simulink model "LKAS_AutoSave_DF_20220125_0841"  (R2018b)
settings: Solver=FixedStepDiscrete  StartTime=0.0  StopTime=10.0  FixedStep=0.01  RelTol=1e-3
InitFcn:
  | tmpVer = ver('MATLAB');
  | tmpVer = str2num(tmpVer.Version);
  | % -------------------------------------------------------------------
  | %  MATLAB file generated by Simulink.saveVars on 21-Nov-2019 10:06:14
  | %  MATLAB version: 7.13.0.564 (R2011b)
  | % -------------------------------------------------------------------
  | 
  | 
  | SInt16 = Simulink.AliasType;
  | SInt16.Description = 'Num';
  | if (tmpVer > 7.11)
  | 	SInt16.DataScope = 'Auto';
  | end
  | SInt16.HeaderFile = 'Rte_Type.h';
  | SInt16.BaseType = 'int16';
  | 
  | SInt32 = Simulink.AliasType;
  | SInt32.Description = 'Num';
  | if (tmpVer > 7.11)
  | 	SInt32.DataScope = 'Auto';
  | end
  | SInt32.HeaderFile = 'Rte_Type.h';
  | SInt32.BaseType = 'int32';
  | 
  | SInt8 = Simulink.AliasType;
  | SInt8.Description = 'Num';
  | if (tmpVer > 7.11)
  | 	SInt8.DataScope = 'Auto';
  | end
  | SInt8.HeaderFile = 'Rte_Type.h';
  | SInt8.BaseType = 'int8';
  | 
  | T_A_m2_1024_1_u32 = Simulink.NumericType;
  | T_A_m2_1024_1_u32.Description = 'm2 (square meters  (m2))';
  | if (tmpVer > 7.11)
  | 	T_A_m2_1024_1_u32.DataScope = 'Auto';
  | end
  | T_A_m2_1024_1_u32.HeaderFile = 'Rte_Type.h';
  | T_A_m2_1024_1_u32.DataTypeMode = 'Fixed-point: slope and bias scaling';
  | T_A_m2_1024_1_u32.SignednessBool = false;
  | T_A_m2_1024_1_u32.WordLength = 32;
  | T_A_m2_1024_1_u32.FixedExponent = -10;
  | T_A_m2_1024_1_u32.SlopeAdjustmentFactor = 1;
  | T_A_m2_1024_1_u32.Bias = 0;
  | T_A_m2_1024_1_u32.DataTypeOverride = 'Inherit';
  | T_A_m2_1024_1_u32.IsAlias = true;
  | 
  | T_A_m2_65536_1_u16 = Simulink.NumericType;
  | T_A_m2_65536_1_u16.Description = 'm2 (square meters  (m2))';
  | if (tmpVer > 7.11)
  | 	T_A_m2_65536_1_u16.DataScope = 'Auto';
  | end
  | T_A_m2_65536_1_u16.HeaderFile = 'Rte_Type.h';
  | T_A_m2_65536_1_u16.DataTypeMode = 'Fixed-point: slope and bias scaling';
  | T_A_m2_65536_1_u16.SignednessBool = false;
  | T_A_m2_65536_1_u16.WordLength = 16;
  | T_A_m2_65536_1_u16.FixedExponent = -16;
  | T_A_m2_65536_1_u16.SlopeAdjustmentFactor = 1;
  | T_A_m2_65536_1_u16.Bias = 0;
  | T_A_m2_65536_1_u16.DataTypeOverride = 'Inherit';
  | ... (+4647 lines)
StopFcn:
  | clear  T_A_m2_1024_1_u32 T_A_m2_65536_1_u16 T_A_m2_Float32 T_A_mm2_10_1_u16 T_A_mm2_4_1_s16 T_A_mm2_Float32 T_Cnt_Num_10_1_u32 T_Cnt_Num_1_1_s16 T_Cnt_Num_1_1_s32 T_Cnt_Num_1_1_s8 T_Cnt_Num_1_1_u16 T_Cnt_Num_1_1_u32 T_Cnt_Num_1_1_u8 T_E_J_1_1_s32 T_E_J_Float32 T_E_kJ_128_1_s32 T_E_kJ_Float32 T_E_kwh_10_1_u16 T_E_kwh_Float32 T_Epl_kwhpkm_100_1_u16 T_Epl_kwhpkm_Float32 T_F_N_1_1_s16 T_F_N_Float32 T_I_A_1000_1_u16 T_I_A_1048576_1_s32 T_I_A_2048_1_s16 T_I_A_32_1_s16 T_I_A_Float32 T_I_mA_1_1_s16 T_I_mA_32768_128_s16 T_I_mA_Float32 T_J_kgpm2_128_1_u16 T_J_kgpm2_Float32 T_K_NA_1000_1_s16 T_K_NA_100_1_s16 T_K_NA_100_1_u16 T_K_NA_1024_1_s16 T_K_NA_1024_1_u16 T_K_NA_128_1_s16 T_K_NA_128_1_u16 T_K_NA_128_1_u8 T_K_NA_16777216_1_u32 T_K_NA_16_1_s16 T_K_NA_16_1_u16 T_K_NA_16_1_u8 T_K_NA_1_16_u16 T_K_NA_1_1_s16 T_K_NA_1_1_u16 T_K_NA_1_1_u8 T_K_NA_32768_1_s16 T_K_NA_32768_1_u16 T_K_NA_32_1_s8 T_K_NA_4096_1_u16 T_K_NA_4194304_1_s32 T_K_NA_4194304_1_u16 T_K_NA_65536_1_s32 T_K_NA_65536_1_u16 T_K_NA_8192_1_s16 T_K_NA_8_1_s16 T_K_NA_Float32 T_M_Nm_16_1_s16 T_M_Nm_1_1_s16 T_M_Nm_32768_1_s16 T_M_Nm_32_1_s16 T_M_Nm_4_1_s16 T_M_Nm_512_1_s16 T_M_Nm_Float32 T_P_W_1_4_s16 T_P_W_1_8_s16 T_P_W_Float32 T_P_kW_128_1_s16 T_P_kW_1_8_s16 T_P_kW_8_1_s32 T_P_kW_Float32 T_Pct_pct_1024_1_s32 T_Pct_pct_1024_1_u32 T_Pct_pct_10_1_s16 T_Pct_pct_10_1_u32 T_Pct_pct_128_100_s8 T_Pct_pct_1_1_s16 T_Pct_pct_1_4_u8 T_Pct_pct_255_100_u16 T_Pct_pct_255_100_u8 T_Pct_pct_256_1_s16 T_Pct_pct_256_1_u16 T_Pct_pct_65535_100_u16 T_Pct_pct_Float32 T_R_ohm_1024_1_s16 T_R_ohm_32_1_s16 T_R_ohm_Float32 T_TK_K_16_1_s16 T_TK_K_Float32 T_T_degC_10_400_1_u16 T_T_degC_16_1_s16 T_T_degC_1_40_1_u8 T_T_degC_2_80_1_u8 T_T_degC_Float32 T_U_V_1000_1_u16 T_U_V_10_1_u8 T_U_V_200_1_u8 T_U_V_32_1_s16 T_U_V_4096_1_s16 T_U_V_512_1_s16 T_U_V_65535_8_u16 T_U_V_8192_1_u16 T_U_V_Float32 T_U_mV_1_1_s16 T_U_mV_256_20_u16 T_U_mV_Float32 T_V_l_256_1_s16 T_V_l_4096_1_s16 T_V_l_64_1_s16 T_V_l_65535_100_u16 T_V_l_Float32 T_V_ml_128_1_s16 T_V_ml_1_1_s16 T_V_ml_32768_1_s16 T_V_ml_Float32 T_V_ul_32_1_u16 T_V_ul_Float32 T_Vpl_clpkm_512_1_u16 T_Vpl_clpkm_Float32 T_a_kphps_16_1_s16 T_a_kphps_Float32 T_a_mps2_128_1_s16 T_a_mps2_Float32 T_c_MJpkg_256_1_s16 T_c_MJpkg_Float32 T_c_kJpgpK_1024_1_s16 T_c_kJpgpK_Float32 T_c_kJpkgpK_128_1_u16 T_c_kJpkgpK_Float32 T_chrg_Ah_1_1_s16 T_chrg_Ah_1_1_u16 T_chrg_Ah_1_1_u8 T_chrg_Ah_256_1_u16 T_chrg_Ah_4194304_1_s32 T_chrg_Ah_512_1_u16 T_chrg_Ah_8_1_u16 T_chrg_Ah_Float32 T_cmp_NA_100_1_s16 T_cmp_NA_128_1_s16 T_cmp_NA_16_1_s16 T_cmp_NA_32768_1_u16 T_cmp_NA_Float32 T_d2n_rpmps2_4_1_s16 T_d2n_rpmps2_Float32 T_dPct_pctps_16_1_s16 T_dPct_pctps_256_1_s16 T_dPct_pctps_Float32 T_dT_degCps_128_1_s16 T_dT_degCps_Float32 T_dV_lph_1_1_s16 T_dV_lph_Float32 T_dV_lpm_128_1_s16 T_dV_lpm_32_1_s16 T_dV_lpm_Float32 T_dV_lps_1024_1_u16 T_dV_lps_4_1_u16 T_dV_lps_Float32 T_dV_mlps_1024_1_s16 T_dV_mlps_Float32 T_d_BitField16 T_dm_gps_128_1_s16 T_dm_gps_128_1_u16 T_dm_gps_256_1_u16 T_dm_gps_Float32 T_dm_mgps_1_1_s16 T_dm_mgps_Float32 T_dn_rpmps_1_1_s16 T_dn_rpmps_2_1_s16 T_dn_rpmps_Float32 T_dp_Paps_1_1_s16 T_dp_Paps_Float32 T_dp_kPaps_1_1_s16 T_dp_kPaps_8_1_s16 T_dp_kPaps_Float32 T_dphi_degps_128_1_s16 T_dphi_degps_8_1_s16 T_dphi_degps_Float32 T_dr_ps_256_1_s16 T_dr_ps_Float32 T_drho_mgplps_1_2_s16 T_drho_mgplps_Float32 T_e_NA_1_1_u8 T_f_Hz_1_1_u16 T_f_Hz_1_1_u32 T_f_Hz_64_1_u16 T_f_Hz_8_1_s16 T_f_Hz_Float32 T_g_BitField32 T_l_km_16_1_s16 T_l_km_1_1_u16 T_l_km_1_1_u32 T_l_km_Float32 T_l_m_1024_1_s16 T_l_m_16_1_s16 T_l_m_1_1_u32 T_l_m_Float32 T_l_mm_16_1_s16 T_l_mm_1_1_u16 T_l_mm_4096_1_s16 T_l_mm_4_1_u8 T_l_mm_64_1_s16 T_l_mm_Float32 T_m_g_1_1_s16 T_m_g_2048_1_s16 T_m_g_32_1_u16 T_m_g_Float32 T_m_kg_1024_1_s16 T_m_kg_1_1_s16 T_m_kg_1_1_u32 T_m_kg_Float32 T_m_mg_128_1_s16 T_m_mg_32_1_s16 T_m_mg_Float32 T_n_rpm_1_1_s16 T_n_rpm_1_25_u8 T_n_rpm_256_50_u16 T_n_rpm_2_25_u8 T_n_rpm_4_1_u16 T_n_rpm_Float32 T_p_MPa_64_1_s16 T_p_MPa_Float32 T_p_Pa_1_1_s16 T_p_Pa_Float32 T_p_kPa_1_10_u16 T_p_kPa_1_1_s16 T_p_kPa_1_1_u8 T_p_kPa_256_1_u16 T_p_kPa_32_1_u16 T_p_kPa_64_1_s16 T_p_kPa_Float32 T_phi_deg_100_1_s16 T_phi_deg_1024_1_s16 T_phi_deg_128_1_s16 T_phi_deg_1_1_u8 T_phi_deg_256_1_s16 T_phi_deg_2_1_s8 T_phi_deg_32_1_s16 T_phi_deg_512_6_s32 T_phi_deg_Float32 T_phi_rad_2048_1_s16 T_phi_rad_Float32 T_r_NA_1024_1_s16 T_r_NA_1024_1_u16 T_r_NA_16384_1_s16 T_r_NA_16_1_s16 T_r_NA_256_1_s8 T_r_NA_256_1_u16 T_r_NA_32768_1_u16 T_r_NA_32_1_u16 T_r_NA_4096_1_s16 T_r_NA_65535_2_u16 T_r_NA_8192_1_u16 T_r_NA_Float32 T_rho_gpl_8192_1_s16 T_rho_gpl_Float32 T_rho_kgpm3_16_1_s16 T_rho_kgpm3_Float32 T_rho_mgpl_1_1_s16 T_rho_mgpl_64_1_s16 T_rho_mgpl_Float32 T_t_hour_1_1_s16 T_t_hour_Float32 T_t_m_1_1_u16 T_t_m_Float32 T_t_ms_1_1_s16 T_t_ms_1_1_u16 T_t_ms_1_1_u32 T_t_ms_4096_1_s16 T_t_ms_64_1_s16 T_t_ms_Float32 T_t_s_1000_1_s16 T_t_s_100_1_s16 T_t_s_10_1_s16 T_t_s_10_1_u16 T_t_s_1_1_s16 T_t_s_1_1_u16 T_t_s_1_1_u32 T_t_s_Float32 T_t_us_10_1_u32 T_t_us_1_1_s16 T_t_us_1_1_u32 T_t_us_1_4_u16 T_t_us_Float32 T_v_kph_1_1_u8 T_v_kph_64_1_s16 T_v_kph_64_1_u16 T_v_kph_Float32 T_v_mps_256_1_s16 T_v_mps_Float32 T_w_radps_32_1_s16 T_w_radps_Float32 T_y_BitField8 T_y_BitFieldDiagProgress T_y_BitFieldDiagStatus T_y_NA_1_1_u8 SInt16 SInt32 SInt8 T_BOOLEAN UInt16 UInt32 UInt8 s16 s32 s8 u16 u32 u8
model workspace (MAT data in the model file):
  MCOS : class17 (value not decoded)
  MCOS : class17 (value not decoded)
  MCOS : class17 (value not decoded)
  MCOS : class17 (value not decoded)
  MCOS : class17 (value not decoded)
  MCOS : class17 (value not decoded)
  MCOS : class17 (value not decoded)
  MCOS : class17 (value not decoded)
  MCOS : class17 (value not decoded)
  MCOS : class17 (value not decoded)
  MCOS : class17 (value not decoded)
  MCOS : class17 (value not decoded)
  MCOS : class17 (value not decoded)
  MCOS : class17 (value not decoded)
  MCOS : class17 (value not decoded)
  MCOS : class17 (value not decoded)
  MCOS : class17 (value not decoded)
  MCOS : class17 (value not decoded)
  MCOS : class17 (value not decoded)
  MCOS : class17 (value not decoded)
  MCOS : class17 (value not decoded)
  MCOS : class17 (value not decoded)
  MCOS : class17 (value not decoded)
  MCOS : class17 (value not decoded)
  MCOS : class17 (value not decoded)
  MCOS : class17 (value not decoded)
  MCOS : class17 (value not decoded)
  MCOS : class17 (value not decoded)
  MCOS : class17 (value not decoded)
  MCOS : class17 (value not decoded)
  MCOS : class17 (value not decoded)
  MCOS : class17 (value not decoded)
  MCOS : class17 (value not decoded)
  MCOS : class17 (value not decoded)
  MCOS : class17 (value not decoded)
  MCOS : class17 (value not decoded)
  MCOS : class17 (value not decoded)
  MCOS : class17 (value not decoded)
  MCOS : class17 (value not decoded)
  MCOS : class17 (value not decoded)
  MCOS : class17 (value not decoded)
  MCOS : class17 (value not decoded)
  MCOS : class17 (value not decoded)
  MCOS : class17 (value not decoded)
  MCOS : class17 (value not decoded)
  MCOS : class17 (value not decoded)
  MCOS : class17 (value not decoded)
  MCOS : class17 (value not decoded)
  MCOS : class17 (value not decoded)
  MCOS : class17 (value not decoded)
  MCOS : class17 (value not decoded)
  MCOS : class17 (value not decoded)
  MCOS : class17 (value not decoded)
  MCOS : class17 (value not decoded)
  MCOS : class17 (value not decoded)
  MCOS : class17 (value not decoded)
  MCOS : class17 (value not decoded)
  MCOS : class17 (value not decoded)
  MCOS : class17 (value not decoded)
  MCOS : class17 (value not decoded)
  MCOS : class17 (value not decoded)
  MCOS : class17 (value not decoded)
  MCOS : class17 (value not decoded)
  MCOS : class17 (value not decoded)
  MCOS : class17 (value not decoded)
  MCOS : class17 (value not decoded)
  MCOS : class17 (value not decoded)
  MCOS : class17 (value not decoded)
  MCOS : class17 (value not decoded)
  MCOS : class17 (value not decoded)
  MCOS : class17 (value not decoded)
  MCOS : class17 (value not decoded)
  MCOS : class17 (value not decoded)
  MCOS : class17 (value not decoded)
  MCOS : class17 (value not decoded)
  MCOS : class17 (value not decoded)
  MCOS : class17 (value not decoded)
  MCOS : class17 (value not decoded)
  MCOS : class17 (value not decoded)
  MCOS : class17 (value not decoded)
  MCOS : class17 (value not decoded)
  MCOS : class17 (value not decoded)
  MCOS : class17 (value not decoded)
  MCOS : class17 (value not decoded)
  MCOS : class17 (value not decoded)
  MCOS : class17 (value not decoded)
  MCOS : class17 (value not decoded)
  MCOS : class17 (value not decoded)
  MCOS : class17 (value not decoded)
  MCOS : class17 (value not decoded)
  MCOS : class17 (value not decoded)
  MCOS : class17 (value not decoded)
  MCOS : class17 (value not decoded)
  MCOS : class17 (value not decoded)
  MCOS : class17 (value not decoded)
  MCOS : class17 (value not decoded)
  MCOS : class17 (value not decoded)
  MCOS : class17 (value not decoded)
  MCOS : class17 (value not decoded)
  MCOS : class17 (value not decoded)
  MCOS : class17 (value not decoded)
  MCOS : class17 (value not decoded)
undefined symbols (not defined in the file): LKA_CarWidth, LKA_SampleTime, LKA_StrRatio_C, LKA_Veh2CamL_C, LKA_Veh2CamW_C, LKA_WhlBaseL_C, LL_CompHdAg_C, LL_CompSWA_C, LL_CrvtPrvwT_C, LL_DesDvt_C, LL_DvtComp_C, LL_DvtPrvwT_C, LL_DvtSpdDet_vDvtSpdMin_C, LL_HandsOff_ExitTime, LL_HandsOff_TextTime, LL_HandsOff_WarnTime, LL_HdAgExT_C, LL_HdAgPrvwT_C, LL_LAccMax_C, LL_LAccRMax_C, LL_LDW_EarliestWarnLine_C, LL_LDW_LatestWarnLine_C, LL_LDWS_SUPPRESS_HEADING, LL_LFClb_TFC_FfCtlRatio_C, LL_LFClb_TFC_KdBalance_C, LL_LFClb_TFC_KdMaxSWA_C, LL_LFClb_TFC_KdV1_C, LL_LFClb_TFC_KdV2_C, LL_LFClb_TFC_KdVehSpdLwr_C, LL_LFClb_TFC_KdVehSpdUpr_C, LL_LFClb_TFC_Ki_C, LL_LFClb_TFC_KiMaxSWA_C, LL_LFClb_TFC_Kp_C, LL_LFClb_TFC_KpKlat_C, LL_LFClb_TFC_KpV1_C, LL_LFClb_TFC_KpV2_C, LL_LFClb_TFC_KpVehSpdLwr_C, LL_LFClb_TFC_KpVehSpdUpr_C, LL_LFClb_TFC_PrvwT_C, LL_LKA_EarliestWarnLine_C, LL_LKA_LatestWarnLine_C, LL_LKAExPrcs_ExitC0Dvt, LL_LKAExPrcs_ExitC0Swt, LL_LKAExPrcs_tiExitTime1, LL_LKAExPrcs_tiExitTime2, LL_LKAExPrcs_tiExitTime3, LL_LKAS_OUT_OF_CONTROL_LAT_VEL, LL_LKAS_OUT_OF_CONTROL_TTLC, LL_LKASWASyn_M0, LL_LKASWASyn_M1, LL_LKASWASyn_M2, LL_LKASWASyn_M3K, LL_LKASWASyn_SWAaddMax, LL_LKASWASyn_T2, LL_LKASWASyn_tiTrqSwaRtTime, LL_LKASWASyn_tiTrqSwaTime, LL_LKASWASyn_TrqMax, LL_LKASWASyn_TrqSwaAddSwt, LL_LKASWASyn_TrqSwaRateDiff, LL_LSpdCompT_C ... (+43)
libraries: simulink x136, canmsglib x8, dspstat3 x3, simulink_extras x1
(part 5 of 20)

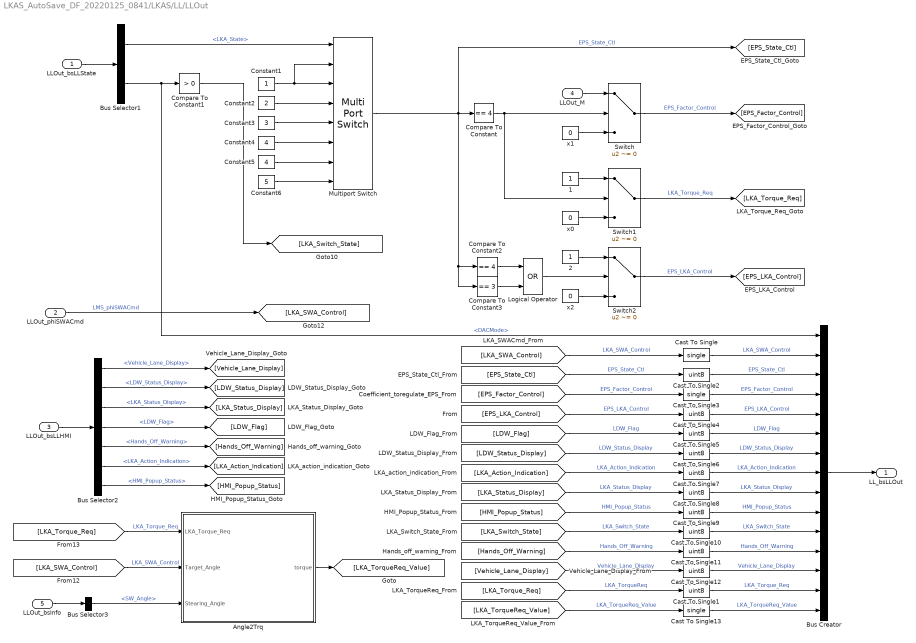
== system LKAS_AutoSave_DF_20220125_0841/LKAS/LL/LLOut ==
  LLOut_bsLLState : Inport
  LLOut_phiSWACmd : Inport  Port=2
  LLOut_bsLLHMI : Inport  Port=3
  LLOut_M : Inport  Port=4
  LLOut_bsInfo : Inport  Port=5
  1 : Constant  OutDataTypeStr=uint8
      settings: AttributesFormatString=DT: %<OutDataTypeStr>
  2 : Constant  OutDataTypeStr=uint8
      settings: AttributesFormatString=DT: %<OutDataTypeStr>
  Angle2Trq : Subsystem
  Bus Creator : BusCreator  Inputs=15
  Bus Selector1 : BusSelector  OutputSignals=LKA_State,DACMode
  Bus Selector2 : BusSelector  OutputSignals=Vehicle_Lane_Display,LDW_Status_Display,LKA_Status_Display,LDW_Flag,Hands_Off_Warning,LKA_Action_Indication,HMI_Popup_Status
  Bus Selector3 : BusSelector  OutputSignals=bsSWAInfo.SW_Angle
  Cast To Single : DataTypeConversion  OutDataTypeStr=single
  Cast To Single{1..2,4..12} (11 alike) : DataTypeConversion  OutDataTypeStr=uint8
  Cast To Single13 : DataTypeConversion  OutDataTypeStr=single
  Cast To Single3 : DataTypeConversion  OutDataTypeStr=single
  Compare To Constant : simulink/Logic and Bit Operations/Compare To Constant  relop===  const=4  OutDataTypeStr=boolean
  Compare To Constant1 : simulink/Logic and Bit Operations/Compare To Constant  relop=>  const=0  OutDataTypeStr=boolean
  Compare To Constant2 : simulink/Logic and Bit Operations/Compare To Constant  relop===  const=4  OutDataTypeStr=boolean
  Compare To Constant3 : simulink/Logic and Bit Operations/Compare To Constant  relop===  const=3  OutDataTypeStr=boolean
  Constant1 : Constant  OutDataTypeStr=uint8
  Constant2 : Constant  Value=2  OutDataTypeStr=uint8
  Constant3 : Constant  Value=3  OutDataTypeStr=uint8
  Constant4 : Constant  Value=4  OutDataTypeStr=uint8
  Constant5 : Constant  Value=4  OutDataTypeStr=uint8
  Constant6 : Constant  Value=5  OutDataTypeStr=uint8
  Logical Operator : Logic  Operator=OR  AllPortsSameDT=off  OutDataTypeStr=boolean
  Multiport Switch : MultiPortSwitch  DataPortOrder=Zero-based contiguous  Inputs=7  zeroidx=on
  Switch : Switch  Criteria=u2 ~= 0
      settings: AttributesFormatString=%<Criteria>
  Switch1 : Switch  Criteria=u2 ~= 0
      settings: AttributesFormatString=%<Criteria>
  Switch2 : Switch  Criteria=u2 ~= 0
      settings: AttributesFormatString=%<Criteria>
  x0 : Constant  Value=0  OutDataTypeStr=uint8
      settings: AttributesFormatString=DT: %<OutDataTypeStr>
  x1 : Constant  Value=0  OutDataTypeStr=uint8
      settings: AttributesFormatString=DT: %<OutDataTypeStr>
  x2 : Constant  Value=0  OutDataTypeStr=uint8
      settings: AttributesFormatString=DT: %<OutDataTypeStr>
  LL_bsLLOut : Outport
      settings: AttributesFormatString=Disable Action: %<OutputWhenDisabled>
  wires:
  Cast To Single13/1 -> Bus Creator/15  "LKA_TorqueReq_Value"
  [LKA_TorqueReq_Value] -> Cast To Single13/1  "LKA_TorqueReq_Value"
  Cast To Single1/1 -> Bus Creator/14  "LKA_Torque_Req"
  [LKA_Torque_Req] -> Cast To Single1/1  "LKA_TorqueReq"
  Cast To Single7/1 -> Bus Creator/8  "LKA_Action_Indication"
  Compare To Constant/1 -> Switch/2, Switch1/2
  [Vehicle_Lane_Display] -> Cast To Single12/1  "Vehicle_Lane_Display"
  [EPS_LKA_Control] -> Cast To Single4/1  "EPS_LKA_Control"
  [LDW_Flag] -> Cast To Single5/1  "LDW_Flag"
  [EPS_Factor_Control] -> Cast To Single3/1  "EPS_Factor_Control"
  [LKA_Action_Indication] -> Cast To Single7/1  "LKA_Action_Indication"
  Constant6/1 -> Multiport Switch/8
  Cast To Single5/1 -> Bus Creator/6  "LDW_Flag"
  [HMI_Popup_Status] -> Cast To Single9/1  "HMI_Popup_Status"
  Bus Selector1/1 -> Multiport Switch/1  "<LKA_State>"
  [LKA_Status_Display] -> Cast To Single8/1  "LKA_Status_Display"
  [LKA_SWA_Control] -> Cast To Single/1  "LKA_SWA_Control"
  Cast To Single/1 -> Bus Creator/2  "LKA_SWA_Control"
  [LDW_Status_Display] -> Cast To Single6/1  "LDW_Status_Display"
  [LKA_Switch_State] -> Cast To Single10/1  "LKA_Switch_State"
  [Hands_Off_Warning] -> Cast To Single11/1  "Hands_Off_Warning"
  Cast To Single8/1 -> Bus Creator/9  "LKA_Status_Display"
  Cast To Single4/1 -> Bus Creator/5  "EPS_LKA_Control"
  Cast To Single10/1 -> Bus Creator/11  "LKA_Switch_State"
  Bus Selector1/2 -> Bus Creator/1, Compare To Constant1/1  "<DACMode>"
  Constant2/1 -> Multiport Switch/4
  Cast To Single2/1 -> Bus Creator/3  "EPS_State_Ctl"
  Bus Creator/1 -> LL_bsLLOut/1
  Cast To Single3/1 -> Bus Creator/4  "EPS_Factor_Control"
  Constant3/1 -> Multiport Switch/5
  Multiport Switch/1 -> Compare To Constant2/1, Compare To Constant3/1, [EPS_State_Ctl], Compare To Constant/1  "EPS_State_Ctl"
  Switch/1 -> [EPS_Factor_Control]  "EPS_Factor_Control"
  Cast To Single6/1 -> Bus Creator/7  "LDW_Status_Display"
  Cast To Single12/1 -> Bus Creator/13  "Vehicle_Lane_Display"
  [EPS_State_Ctl] -> Cast To Single2/1  "EPS_State_Ctl"
  LLOut_bsLLState/1 -> Bus Selector1/1
  Compare To Constant1/1 -> [LKA_Switch_State]
  Constant4/1 -> Multiport Switch/6
  Cast To Single9/1 -> Bus Creator/10  "HMI_Popup_Status"
  LLOut_M/1 -> Switch/1
  Cast To Single11/1 -> Bus Creator/12  "Hands_Off_Warning"
  Constant5/1 -> Multiport Switch/7
  Constant1/1 -> Multiport Switch/2, Multiport Switch/3
  Bus Selector2/5 -> [Hands_Off_Warning]  "<Hands_Off_Warning>"
  Bus Selector2/6 -> [LKA_Action_Indication]  "<LKA_Action_Indication>"
  Bus Selector2/2 -> [LDW_Status_Display]  "<LDW_Status_Display>"
  LLOut_bsLLHMI/1 -> Bus Selector2/1
  Bus Selector2/4 -> [LDW_Flag]  "<LDW_Flag>"
  Bus Selector2/3 -> [LKA_Status_Display]  "<LKA_Status_Display>"
  Bus Selector2/7 -> [HMI_Popup_Status]  "<HMI_Popup_Status>"
  Bus Selector2/1 -> [Vehicle_Lane_Display]  "<Vehicle_Lane_Display>"
  Switch1/1 -> [LKA_Torque_Req]  "LKA_Torque_Req"
  1/1 -> Switch1/1
  x0/1 -> Switch1/3
  LLOut_phiSWACmd/1 -> [LKA_SWA_Control]  "LMS_phiSWACmd"
  [LKA_Torque_Req] -> Angle2Trq/1(LKA_Torque_Req)  "LKA_Torque_Req"
  [LKA_SWA_Control] -> Angle2Trq/2(Target_Angle)  "LKA_SWA_Control"
  Angle2Trq/1(torque) -> [LKA_TorqueReq_Value]
  LLOut_bsInfo/1 -> Bus Selector3/1
  Bus Selector3/1 -> Angle2Trq/3(Stearing_Angle)  "<SW_Angle>"
  x1/1 -> Switch/3
  Compare To Constant2/1 -> Logical Operator/1
  Compare To Constant3/1 -> Logical Operator/2
  Logical Operator/1 -> Switch2/2
  Switch2/1 -> [EPS_LKA_Control]  "EPS_LKA_Control"
  2/1 -> Switch2/1
  x2/1 -> Switch2/3

== system LKAS_AutoSave_DF_20220125_0841/LKAS/LLClb/ConstantClb ==
  Bus Creator : BusCreator  Inputs=6
  Data Type Conversion{2..4,6,13,22} (6 alike) : DataTypeConversion  OutDataTypeStr=single
  LKA_CarWidth=1.8 : Constant  Value=LKA_CarWidth
  LKA_SampleTime=0.01 : Constant  Value=LKA_SampleTime  OutDataTypeStr=single
  LKA_StrRatio_C=15.3 : Constant  Value=LKA_StrRatio_C
  LKA_Veh2CamL_C=1.56 : Constant  Value=LKA_Veh2CamL_C
  LKA_Veh2CamW_C=0.9 : Constant  Value=LKA_Veh2CamW_C  OutDataTypeStr=single
  LKA_WhlBaseL_C=2.65 : Constant  Value=LKA_WhlBaseL_C
  Switch{,1..3,11,19} (6 alike) : Switch  Criteria=u2 ~= 0  OutDataTypeStr=single
  ConstantClb : Outport
  wires:
  LKA_SampleTime=0.01/1 -> Switch19/3  "LKA_SampleTime"
  Data Type Conversion3/1 -> Switch19/1, Switch19/2
  Switch19/1 -> Bus Creator/1  "LKA_SampleTime"
  Switch2/1 -> Bus Creator/4  "LKA_WhlBaseL_C"
  Switch/1 -> Bus Creator/2  "LKA_Veh2CamW_C"
  Switch1/1 -> Bus Creator/3  "LKA_Veh2CamL_C"
  Switch11/1 -> Bus Creator/6  "LKA_CarWidth"
  Switch3/1 -> Bus Creator/5  "LKA_StrRatio_C"
  Bus Creator/1 -> ConstantClb/1
  LKA_CarWidth=1.8/1 -> Switch11/3  "LKA_CarWidth"
  Data Type Conversion22/1 -> Switch11/2, Switch11/1
  LKA_StrRatio_C=15.3/1 -> Switch3/3  "LKA_StrRatio_C"
  Data Type Conversion6/1 -> Switch3/2, Switch3/1
  Data Type Conversion4/1 -> Switch2/2, Switch2/1
  LKA_WhlBaseL_C=2.65/1 -> Switch2/3  "LKA_WhlBaseL_C"
  LKA_Veh2CamL_C=1.56/1 -> Switch1/3  "LKA_Veh2CamL_C"
  Data Type Conversion2/1 -> Switch1/2, Switch1/1
  Data Type Conversion13/1 -> Switch/2, Switch/1
  LKA_Veh2CamW_C=0.9/1 -> Switch/3  "LKA_Veh2CamW_C"

== system LKAS_AutoSave_DF_20220125_0841/LKAS/LLClb/LDWClb ==
  Bus Creator : BusCreator  Inputs=1
  Data Type Conversion6 : DataTypeConversion  OutDataTypeStr=single
  LL_LDWS_SUPPRESS_HEADING=2 : Constant  Value=LL_LDWS_SUPPRESS_HEADING  OutDataTypeStr=single
  Switch2 : Switch  Criteria=u2 ~= 0  OutDataTypeStr=single
  LDWClb : Outport
  wires:
  Data Type Conversion6/1 -> Switch2/2, Switch2/1
  LL_LDWS_SUPPRESS_HEADING=2/1 -> Switch2/3
  Switch2/1 -> Bus Creator/1  "LL_LDWS_SUPPRESS_HEADING"
  Bus Creator/1 -> LDWClb/1

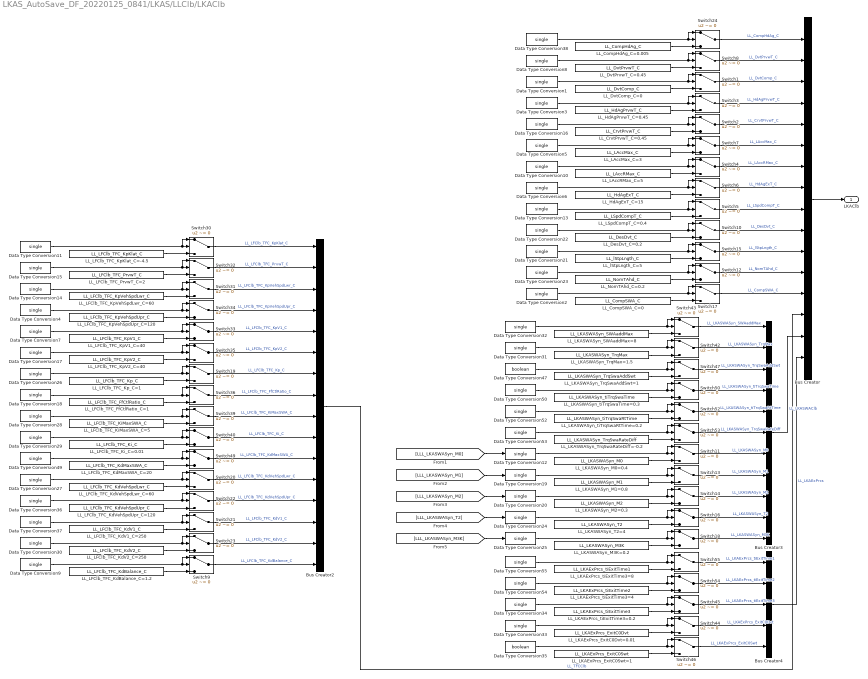
== system LKAS_AutoSave_DF_20220125_0841/LKAS/LLClb/LKAClb ==
  Bus Creator : BusCreator  Inputs=16
  Bus Creator2 : BusCreator  Inputs=16
  Bus Creator3 : BusCreator  Inputs=11
  Bus Creator4 : BusCreator  Inputs=5
  Data Type Conversion{1..34,36..38,49..50,52..55} (43 alike) : DataTypeConversion  OutDataTypeStr=single
  Data Type Conversion35 : DataTypeConversion  OutDataTypeStr=boolean
  Data Type Conversion47 : DataTypeConversion  OutDataTypeStr=boolean
  LL_CompHdAg_C=0.005 : Constant  Value=LL_CompHdAg_C  OutDataTypeStr=single
  LL_CompSWA_C=0 : Constant  Value=LL_CompSWA_C  OutDataTypeStr=single
  LL_CrvtPrvwT_C=0.45 : Constant  Value=LL_CrvtPrvwT_C  OutDataTypeStr=single
  LL_DesDvt_C=0.2 : Constant  Value=LL_DesDvt_C  OutDataTypeStr=single
  LL_DvtComp_C=0 : Constant  Value=LL_DvtComp_C  OutDataTypeStr=single
  LL_DvtPrvwT_C=0.45 : Constant  Value=LL_DvtPrvwT_C  OutDataTypeStr=single
  LL_HdAgExT_C=15 : Constant  Value=LL_HdAgExT_C  OutDataTypeStr=single
  LL_HdAgPrvwT_C=0.45 : Constant  Value=LL_HdAgPrvwT_C  OutDataTypeStr=single
  LL_LAccMax_C=3 : Constant  Value=LL_LAccMax_C  OutDataTypeStr=single
  LL_LAccRMax_C=5 : Constant  Value=LL_LAccRMax_C  OutDataTypeStr=single
  LL_LFClb_TFC_FfCtlRatio_C=1 : Constant  Value=LL_LFClb_TFC_FfCtlRatio_C  OutDataTypeStr=single
  LL_LFClb_TFC_KdBalance_C=1.2 : Constant  Value=LL_LFClb_TFC_KdBalance_C  OutDataTypeStr=single
  LL_LFClb_TFC_KdMaxSWA_C=20 : Constant  Value=LL_LFClb_TFC_KdMaxSWA_C  OutDataTypeStr=single
  LL_LFClb_TFC_KdV1_C=250 : Constant  Value=LL_LFClb_TFC_KdV1_C  OutDataTypeStr=single
  LL_LFClb_TFC_KdV2_C=250 : Constant  Value=LL_LFClb_TFC_KdV2_C  OutDataTypeStr=single
  LL_LFClb_TFC_KdVehSpdLwr_C=60 : Constant  Value=LL_LFClb_TFC_KdVehSpdLwr_C  OutDataTypeStr=single
  LL_LFClb_TFC_KdVehSpdUpr_C=120 : Constant  Value=LL_LFClb_TFC_KdVehSpdUpr_C  OutDataTypeStr=single
  LL_LFClb_TFC_KiMaxSWA_C=5 : Constant  Value=LL_LFClb_TFC_KiMaxSWA_C  OutDataTypeStr=single
  LL_LFClb_TFC_Ki_C=0.01 : Constant  Value=LL_LFClb_TFC_Ki_C  OutDataTypeStr=single
  LL_LFClb_TFC_KpKlat_C=-4.5 : Constant  Value=LL_LFClb_TFC_KpKlat_C  OutDataTypeStr=single
  LL_LFClb_TFC_KpV1_C=40 : Constant  Value=LL_LFClb_TFC_KpV1_C  OutDataTypeStr=single
  LL_LFClb_TFC_KpV2_C=40 : Constant  Value=LL_LFClb_TFC_KpV2_C  OutDataTypeStr=single
  LL_LFClb_TFC_KpVehSpdLwr_C=60 : Constant  Value=LL_LFClb_TFC_KpVehSpdLwr_C  OutDataTypeStr=single
  LL_LFClb_TFC_KpVehSpdUpr_C=120 : Constant  Value=LL_LFClb_TFC_KpVehSpdUpr_C  OutDataTypeStr=single
  LL_LFClb_TFC_Kp_C=1 : Constant  Value=LL_LFClb_TFC_Kp_C  OutDataTypeStr=single
  LL_LFClb_TFC_PrvwT_C=2 : Constant  Value=LL_LFClb_TFC_PrvwT_C  OutDataTypeStr=single
  LL_LKAExPrcs_ExitC0Dvt=0.01 : Constant  Value=LL_LKAExPrcs_ExitC0Dvt  OutDataTypeStr=single
  LL_LKAExPrcs_ExitC0Swt=1 : Constant  Value=LL_LKAExPrcs_ExitC0Swt  OutDataTypeStr=boolean
  LL_LKAExPrcs_tiExitTime3=0.2 : Constant  Value=LL_LKAExPrcs_tiExitTime3  OutDataTypeStr=single
  LL_LKAExPrcs_tiExitTime3=4 : Constant  Value=LL_LKAExPrcs_tiExitTime2  OutDataTypeStr=single
  LL_LKAExPrcs_tiExitTime3=8 : Constant  Value=LL_LKAExPrcs_tiExitTime1  OutDataTypeStr=single
  LL_LKASWASyn_M0=0.4 : Constant  Value=LL_LKASWASyn_M0  OutDataTypeStr=single
  LL_LKASWASyn_M1=0.8 : Constant  Value=LL_LKASWASyn_M1  OutDataTypeStr=single
  LL_LKASWASyn_M2=0.3 : Constant  Value=LL_LKASWASyn_M2  OutDataTypeStr=single
  LL_LKASWASyn_M3K=0.2 : Constant  Value=LL_LKASWASyn_M3K  OutDataTypeStr=single
  LL_LKASWASyn_SWAaddMax=8 : Constant  Value=LL_LKASWASyn_SWAaddMax  OutDataTypeStr=single
  LL_LKASWASyn_T2=4 : Constant  Value=LL_LKASWASyn_T2  OutDataTypeStr=single
  LL_LKASWASyn_TrqMax=1.5 : Constant  Value=LL_LKASWASyn_TrqMax  OutDataTypeStr=single
  LL_LKASWASyn_TrqSwaAddSwt=1 : Constant  Value=LL_LKASWASyn_TrqSwaAddSwt  OutDataTypeStr=boolean
  LL_LKASWASyn_TrqSwaRateDiff=-0.2 : Constant  Value=LL_LKASWASyn_TrqSwaRateDiff  OutDataTypeStr=single
  LL_LKASWASyn_tiTrqSwaRtTime=0.2 : Constant  Value=LL_LKASWASyn_tiTrqSwaRtTime  OutDataTypeStr=single
  LL_LKASWASyn_tiTrqSwaTime=0.3 : Constant  Value=LL_LKASWASyn_tiTrqSwaTime  OutDataTypeStr=single
  LL_LSpdCompT_C=0.4 : Constant  Value=LL_LSpdCompT_C  OutDataTypeStr=single
  LL_NomTAhd_C=0.2 : Constant  Value=LL_NomTAhd_C  OutDataTypeStr=single
  LL_lStpLngth_C=5 : Constant  Value=LL_lStpLngth_C  OutDataTypeStr=single
  Switch{1..24,30..36,39..40,42..45,49..50,52..55} (43 alike) : Switch  Criteria=u2 ~= 0  OutDataTypeStr=single
  Switch46 : Switch  Criteria=u2 ~= 0  OutDataTypeStr=boolean
  Switch47 : Switch  Criteria=u2 ~= 0  OutDataTypeStr=boolean
  LKAClb : Outport
  wires:
  [LLL_LKASWASyn_M3K] -> Data Type Conversion25/1
  Switch18/1 -> Bus Creator3/11  "LL_LKASWASyn_M3K"
  LL_LKASWASyn_M3K=0.2/1 -> Switch18/3
  Data Type Conversion25/1 -> Switch18/1, Switch18/2
  [LLL_LKASWASyn_M0] -> Data Type Conversion12/1
  Switch11/1 -> Bus Creator3/7  "LL_LKASWASyn_M0"
  LL_LKASWASyn_M0=0.4/1 -> Switch11/3
  Data Type Conversion12/1 -> Switch11/1, Switch11/2
  Data Type Conversion19/1 -> Switch13/2, Switch13/1
  LL_LKASWASyn_M1=0.8/1 -> Switch13/3
  Switch13/1 -> Bus Creator3/8  "LL_LKASWASyn_M1"
  [LLL_LKASWASyn_M1] -> Data Type Conversion19/1
  [LLL_LKASWASyn_M2] -> Data Type Conversion20/1
  Switch14/1 -> Bus Creator3/9  "LL_LKASWASyn_M2"
  LL_LKASWASyn_M2=0.3/1 -> Switch14/3
  Data Type Conversion20/1 -> Switch14/1, Switch14/2
  Data Type Conversion24/1 -> Switch16/2, Switch16/1
  LL_LKASWASyn_T2=4/1 -> Switch16/3
  Switch16/1 -> Bus Creator3/10  "LL_LKASWASyn_T2"
  [LLL_LKASWASyn_T2] -> Data Type Conversion24/1
  Data Type Conversion9/1 -> Switch9/2, Switch9/1
  LL_LFClb_TFC_KdBalance_C=1.2/1 -> Switch9/3
  Switch9/1 -> Bus Creator2/16  "LL_LFClb_TFC_KdBalance_C"
  LL_LKAExPrcs_tiExitTime3=8/1 -> Switch55/3
  Data Type Conversion55/1 -> Switch55/1, Switch55/2
  Switch55/1 -> Bus Creator4/1  "LL_LKAExPrcs_tiExitTime1"
  Switch54/1 -> Bus Creator4/2  "LL_LKAExPrcs_tiExitTime2"
  Data Type Conversion54/1 -> Switch54/2, Switch54/1
  LL_LKAExPrcs_tiExitTime3=4/1 -> Switch54/3
  Switch53/1 -> Bus Creator3/6  "LL_LKASWASyn_TrqSwaRateDiff"
  LL_LKASWASyn_TrqSwaRateDiff=-0.2/1 -> Switch53/3
  Data Type Conversion53/1 -> Switch53/1, Switch53/2
  Data Type Conversion52/1 -> Switch52/2, Switch52/1
  LL_LKASWASyn_tiTrqSwaRtTime=0.2/1 -> Switch52/3
  Switch52/1 -> Bus Creator3/5  "LL_LKASWASyn_tiTrqSwaRtTime"
  Switch50/1 -> Bus Creator3/4  "LL_LKASWASyn_tiTrqSwaTime"
  LL_LKASWASyn_tiTrqSwaTime=0.3/1 -> Switch50/3
  Data Type Conversion50/1 -> Switch50/1, Switch50/2
  Data Type Conversion49/1 -> Switch49/2, Switch49/1
  LL_LFClb_TFC_KdMaxSWA_C=20/1 -> Switch49/3
  Switch49/1 -> Bus Creator2/11  "LL_LFClb_TFC_KdMaxSWA_C"
  Data Type Conversion47/1 -> Switch47/2, Switch47/1
  LL_LKASWASyn_TrqSwaAddSwt=1/1 -> Switch47/3
  Switch47/1 -> Bus Creator3/3  "LL_LKASWASyn_TrqSwaAddSwt"
  Switch46/1 -> Bus Creator4/5  "LL_LKAExPrcs_ExitC0Swt"
  LL_LKAExPrcs_ExitC0Swt=1/1 -> Switch46/3
  Data Type Conversion35/1 -> Switch46/1, Switch46/2
  Bus Creator4/1 -> Bus Creator/16  "LL_LKAExPrcs"
  Data Type Conversion33/1 -> Switch44/2, Switch44/1
  LL_LKAExPrcs_ExitC0Dvt=0.01/1 -> Switch44/3
  LL_LKAExPrcs_tiExitTime3=0.2/1 -> Switch45/3
  Data Type Conversion34/1 -> Switch45/1, Switch45/2
  Switch45/1 -> Bus Creator4/3  "LL_LKAExPrcs_tiExitTime3"
  Switch44/1 -> Bus Creator4/4  "LL_LKAExPrcs_ExitC0Dvt"
  Bus Creator3/1 -> Bus Creator/15  "LL_LKASWAClb"
  Switch42/1 -> Bus Creator3/2  "LL_LKASWASyn_TrqMax"
  Switch43/1 -> Bus Creator3/1  "LL_LKASWASyn_SWAaddMax"
  Data Type Conversion32/1 -> Switch43/2, Switch43/1
  LL_LKASWASyn_SWAaddMax=8/1 -> Switch43/3
  LL_LKASWASyn_TrqMax=1.5/1 -> Switch42/3
  Data Type Conversion31/1 -> Switch42/1, Switch42/2
  Data Type Conversion29/1 -> Switch40/2, Switch40/1
  LL_LFClb_TFC_Ki_C=0.01/1 -> Switch40/3
  Data Type Conversion28/1 -> Switch39/2, Switch39/1
  LL_LFClb_TFC_KiMaxSWA_C=5/1 -> Switch39/3
  Switch39/1 -> Bus Creator2/9  "LL_LFClb_TFC_KiMaxSWA_C"
  Switch40/1 -> Bus Creator2/10  "LL_LFClb_TFC_Ki_C"
  Switch36/1 -> Bus Creator2/8  "LL_LFClb_TFC_FfCtlRatio_C"
  Data Type Conversion18/1 -> Switch36/2, Switch36/1
  LL_LFClb_TFC_FfCtlRatio_C=1/1 -> Switch36/3
  LL_LFClb_TFC_KpKlat_C=-4.5/1 -> Switch30/3
  LL_LFClb_TFC_KpVehSpdUpr_C=120/1 -> Switch34/3
  Data Type Conversion14/1 -> Switch31/1, Switch31/2
  LL_LFClb_TFC_KpV2_C=40/1 -> Switch35/3
  Data Type Conversion17/1 -> Switch35/1, Switch35/2
  Data Type Conversion15/1 -> Switch32/1, Switch32/2
  Data Type Conversion4/1 -> Switch34/1, Switch34/2
  Data Type Conversion7/1 -> Switch33/1, Switch33/2
  Data Type Conversion11/1 -> Switch30/1, Switch30/2
  LL_LFClb_TFC_PrvwT_C=2/1 -> Switch32/3
  LL_LFClb_TFC_KpVehSpdLwr_C=60/1 -> Switch31/3
  LL_LFClb_TFC_KpV1_C=40/1 -> Switch33/3
  Switch32/1 -> Bus Creator2/2  "LL_LFClb_TFC_PrvwT_C"
  Switch33/1 -> Bus Creator2/5  "LL_LFClb_TFC_KpV1_C"
  Switch34/1 -> Bus Creator2/4  "LL_LFClb_TFC_KpVehSpdUpr_C"
  Switch31/1 -> Bus Creator2/3  "LL_LFClb_TFC_KpVehSpdLwr_C"
  Switch30/1 -> Bus Creator2/1  "LL_LFClb_TFC_KpKlat_C"
  Switch35/1 -> Bus Creator2/6  "LL_LFClb_TFC_KpV2_C"
  Bus Creator2/1 -> Bus Creator/14  "LL_TFCClb"
  LL_CompSWA_C=0/1 -> Switch17/3
  LL_NomTAhd_C=0.2/1 -> Switch12/3
  LL_lStpLngth_C=5/1 -> Switch15/3
  LL_DesDvt_C=0.2/1 -> Switch10/3
  Data Type Conversion2/1 -> Switch17/1, Switch17/2
  Data Type Conversion22/1 -> Switch10/1, Switch10/2
  Data Type Conversion23/1 -> Switch12/1, Switch12/2
  Data Type Conversion21/1 -> Switch15/1, Switch15/2
  LL_LAccMax_C=3/1 -> Switch7/3
  Data Type Conversion5/1 -> Switch7/1, Switch7/2
  Data Type Conversion10/1 -> Switch4/2, Switch4/1
  LL_LAccRMax_C=5/1 -> Switch4/3
  LL_LSpdCompT_C=0.4/1 -> Switch5/3
  Data Type Conversion13/1 -> Switch5/1, Switch5/2
  Data Type Conversion6/1 -> Switch6/1, Switch6/2
  LL_HdAgExT_C=15/1 -> Switch6/3
  LL_HdAgPrvwT_C=0.45/1 -> Switch3/3
  Data Type Conversion3/1 -> Switch3/1, Switch3/2
  Data Type Conversion16/1 -> Switch2/1, Switch2/2
  LL_CrvtPrvwT_C=0.45/1 -> Switch2/3
  LL_DvtComp_C=0/1 -> Switch1/3
  Data Type Conversion1/1 -> Switch1/1, Switch1/2
  Data Type Conversion8/1 -> Switch8/2, Switch8/1
  LL_DvtPrvwT_C=0.45/1 -> Switch8/3
  Switch12/1 -> Bus Creator/12  "LL_NomTAhd_C"
  Switch10/1 -> Bus Creator/10  "LL_DesDvt_C"
  Switch15/1 -> Bus Creator/11  "LL_lStpLngth_C"
  Switch2/1 -> Bus Creator/5  "LL_CrvtPrvwT_C"
  Switch5/1 -> Bus Creator/9  "LL_LSpdCompT_C"
  Switch4/1 -> Bus Creator/7  "LL_LAccRMax_C"
  Switch7/1 -> Bus Creator/6  "LL_LAccMax_C"
  Switch6/1 -> Bus Creator/8  "LL_HdAgExT_C"
  Switch17/1 -> Bus Creator/13  "LL_CompSWA_C"
  Switch3/1 -> Bus Creator/4  "LL_HdAgPrvwT_C"
  Switch1/1 -> Bus Creator/3  "LL_DvtComp_C"
  Switch8/1 -> Bus Creator/2  "LL_DvtPrvwT_C"
  Bus Creator/1 -> LKAClb/1
  Data Type Conversion26/1 -> Switch19/1, Switch19/2
  Switch19/1 -> Bus Creator2/7  "LL_LFClb_TFC_Kp_C"
  LL_LFClb_TFC_Kp_C=1/1 -> Switch19/3
  Data Type Conversion30/1 -> Switch23/1, Switch23/2
  Switch21/1 -> Bus Creator2/14  "LL_LFClb_TFC_KdV1_C"
  LL_LFClb_TFC_KdVehSpdLwr_C=60/1 -> Switch20/3
  LL_LFClb_TFC_KdV1_C=250/1 -> Switch21/3
  Data Type Conversion36/1 -> Switch22/1, Switch22/2
  Data Type Conversion27/1 -> Switch20/1, Switch20/2
  Switch22/1 -> Bus Creator2/13  "LL_LFClb_TFC_KdVehSpdUpr_C"
  Switch20/1 -> Bus Creator2/12  "LL_LFClb_TFC_KdVehSpdLwr_C"
  LL_LFClb_TFC_KdVehSpdUpr_C=120/1 -> Switch22/3
  Switch23/1 -> Bus Creator2/15  "LL_LFClb_TFC_KdV2_C"
  LL_LFClb_TFC_KdV2_C=250/1 -> Switch23/3
  Data Type Conversion37/1 -> Switch21/1, Switch21/2
  Switch24/1 -> Bus Creator/1  "LL_CompHdAg_C"
  Data Type Conversion38/1 -> Switch24/2, Switch24/1
  LL_CompHdAg_C=0.005/1 -> Switch24/3
